simulink library "experiment_lib2"  (Simulink 8.3)
settings: Solver=ode45  SolverMode=SingleTasking  StartTime=0.0  StopTime=10.0  RelTol=1e-3
values from neighbouring files (symbols this model uses):
  kernel_drift = [0.05 0.05 0.05 0.05]    [Pau_Pol_6_Nodes_4_Perd_0_TxRate_0.01.mat]    (also in llencadora_sim.m = ones(1,num_generators)*0.1-0.05)
  kernel_offset = [0 0 0 0]    [Pau_Pol_6_Nodes_4_Perd_0_TxRate_0.01.mat]    (also in llencadora_sim.m = zeros(1,num_generators))
  LL = [0.000782892151765 0.000588394714514 0.000709966836418 0.00082261967749]    [Pau_Pol_6_Nodes_4_Perd_0_TxRate_0.01.mat]    (also in llencadora_sim.m = minLL+(maxLL-minLL)*rand(1,num_loads))
  Lline = [1.0827664502e-05 1.06430432216e-05 1.0255354423e-05 1.05299829153e-05]    [Pau_Pol_6_Nodes_4_Perd_0_TxRate_0.01.mat]    (also in llencadora_sim.m = minLline+(maxLline-minLline)*rand(1,num_lines))
  RL = [0.345490722943 0.282580500651 0.390474448437 0.324054882207]    [Pau_Pol_6_Nodes_4_Perd_0_TxRate_0.01.mat]    (also in llencadora_sim.m = minRL+(maxRL-minRL)*rand(1,num_loads))
  RLa_pos = 0.45    [Pau_Pol_6_Nodes_4_Perd_0_TxRate_0.01.mat]    (also in llencadora_sim.m = maxRL*ones(1,num_loads_act)*4/tot)
  RLa_pre = 0.21    [Pau_Pol_6_Nodes_4_Perd_0_TxRate_0.01.mat]    (also in llencadora_sim.m = minRL*ones(1,num_loads_act)*4/tot)
  Rline = [0.00149363403679 0.00820725625814 0.00655593060546 0.00272568602759]    [Pau_Pol_6_Nodes_4_Perd_0_TxRate_0.01.mat]    (also in llencadora_sim.m = minRline+(maxRline-minRline)*rand(1,num_lines))
  tL = 5    [Pau_Pol_6_Nodes_4_Perd_0_TxRate_0.01.mat]    (also in llencadora_sim.m = 1e10*ones(1,num_loads_act))
  ts = 0.0001    [Pau_Pol_6_Nodes_4_Perd_0_TxRate_0.01.mat]    (also in dintegral_w_code.m; llencadora_sim.m; processor.m = data.ts)
undefined symbols (not defined in the file or in its folder): CL
libraries: powerlib x17, simulink x1, truetime x1
settings Model: Creator=SEPIC  LastModifiedBy=mvelasco

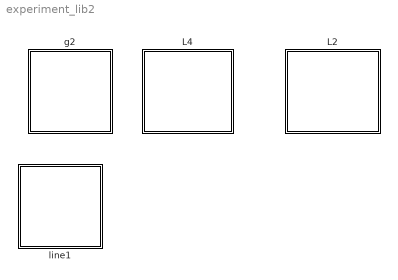
== system experiment_lib2 ==
  L2 : Subsystem  mask{a=1}
      mask Display: disp(['Active\nLoad\n' num2str(a)])
  L4 : Subsystem  mask{a=1}
      mask Display: disp(['Load\nLine\n' num2str(a)])
  g2 : Subsystem  RequirementInfo="{}  %GIDa_067657de_e0d2_47a1_a8cf_e324e59bc421"  mask{a=1}
      mask Display: disp(['Gen\nCom\n' num2str(a)]);
  line1 : Subsystem  mask{a=1}
      mask Display: disp(['Line\n' num2str(a)]);

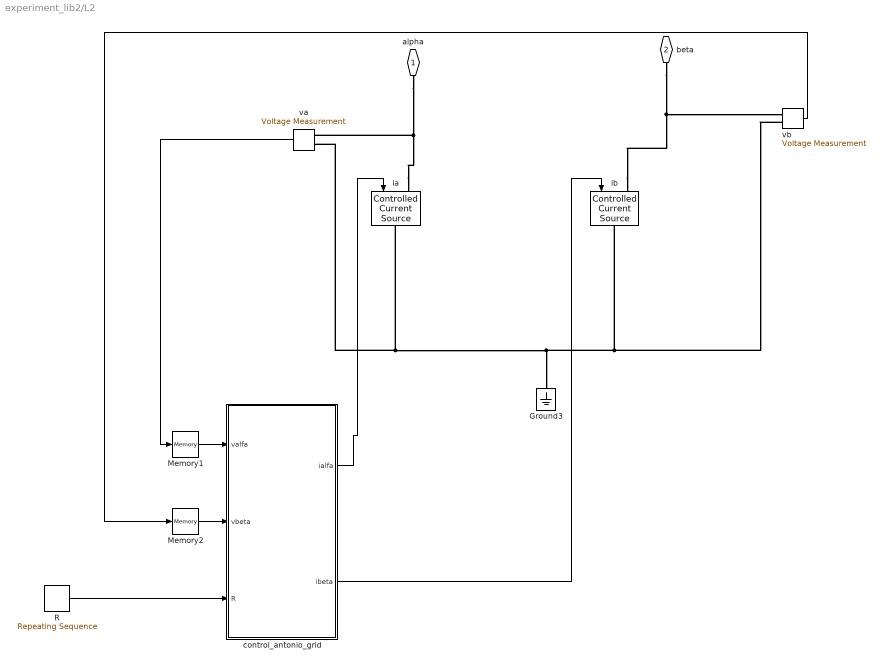
== system experiment_lib2/L2 ==
  Ground3 : powerlib/Elements/Ground  LConnTagsString=a
  Memory1 : Memory
  Memory2 : Memory
  R : simulink/Sources/Repeating Sequence  rep_seq_t=[0 tL(a) tL(a)+ts 1000]  rep_seq_y="[RLa_pre(a)  RLa_pre(a)  RLa_pos(a)  RLa_pos(a) ]"
  control_antonio_grid : MATLAB Function  TreatAsAtomicUnit=on
  ia : powerlib/Electrical Sources/Controlled Current Source  Initialize=on  Source_Type=AC  Amplitude=0  Phase=0  Frequency=0  Measurements=None
  ib : powerlib/Electrical Sources/Controlled Current Source  Initialize=on  Source_Type=AC  Amplitude=0  Phase=0  Frequency=0  Measurements=None
  va : powerlib/Measurements/Voltage Measurement  PhasorSimulation=off  OutputType=Complex  PSBequivalent=0
  vb : powerlib/Measurements/Voltage Measurement  PhasorSimulation=off  OutputType=Complex  PSBequivalent=0
  "alpha " : PMIOPort  Port=1  Side=Left
  beta : PMIOPort  Port=2  Side=Left
  wires:
  R/1 -> control_antonio_grid/3(R)
  va/1 -> Memory1/1
  vb/1 -> Memory2/1
  control_antonio_grid/1(ialfa) -> ia/1
  control_antonio_grid/2(ibeta) -> ib/1
  Memory1/1 -> control_antonio_grid/1(valfa)
  Memory2/1 -> control_antonio_grid/2(vbeta)
  connections:
  vb/LConn2 -- ib/RConn1 -- Ground3/LConn1 -- ia/RConn1 -- va/LConn2
  ia/LConn1 -- "alpha "/RConn1 -- va/LConn1
  ib/LConn1 -- beta/RConn1 -- vb/LConn1

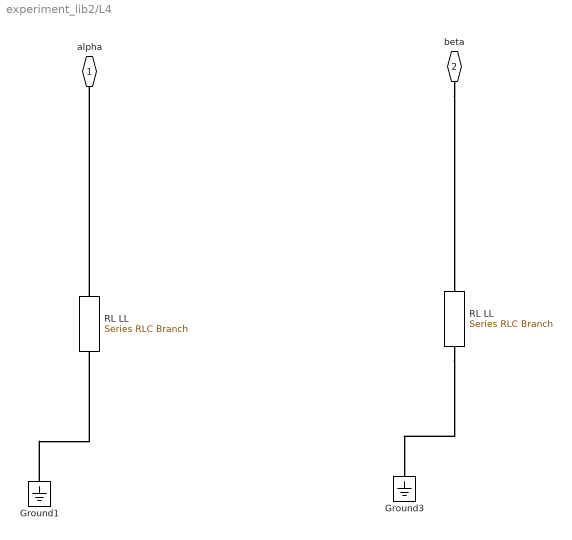
== system experiment_lib2/L4 ==
  Ground1 : powerlib/Elements/Ground  LConnTagsString=a
  Ground3 : powerlib/Elements/Ground  LConnTagsString=a
  RL LL : powerlib/Elements/Series RLC Branch  LConnTagsString=__new0  RConnTagsString=__new0  BranchType=RL  Resistance=RL(a)  Inductance=LL(a)  SetiL0=off  InitialCurrent=0  Capacitance=CL  Setx0=off  InitialVoltage=0  Measurements=None
  "RL LL   " : powerlib/Elements/Series RLC Branch  LConnTagsString=__new0  RConnTagsString=__new0  BranchType=RL  Resistance=RL(a)  Inductance=LL(a)  SetiL0=off  InitialCurrent=0  Capacitance=CL  Setx0=off  InitialVoltage=0  Measurements=None
  "alpha " : PMIOPort  Port=1  Side=Left
  beta : PMIOPort  Port=2  Side=Left
  connections:
  "RL LL   "/RConn1 -- Ground3/LConn1
  beta/RConn1 -- "RL LL   "/LConn1
  Ground1/LConn1 -- RL LL/RConn1
  RL LL/LConn1 -- "alpha "/RConn1

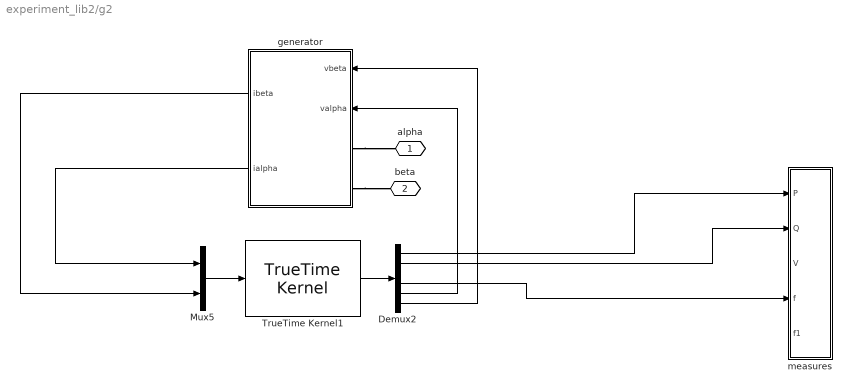
== system experiment_lib2/g2 ==
  Demux2 : Demux  Outputs=6
  Mux5 : Mux  Inputs=2
  TrueTime Kernel1 : truetime/TrueTime Kernel  sfun=kernel_init  args=[a]  ninputsoutputs=[2 6]  ntriggers=0  trigtype=falling  nwnodenbr=[1 a]  clockoffsetdrift=[kernel_offset(a) kernel_drift(a)]  schedoutput=off  battery=off  poweroutput=off
  generator : Subsystem
  measures : Subsystem
  alpha : PMIOPort  Port=1  Side=Left
  beta : PMIOPort  Port=2  Side=Left
  wires:
  generator/2("ialpha ") -> Mux5/1
  generator/1("ibeta ") -> Mux5/2
  Mux5/1 -> TrueTime Kernel1/1
  TrueTime Kernel1/1 -> Demux2/1
  Demux2/6 -> generator/1("vbeta  ")
  Demux2/5 -> generator/2("valpha ")
  Demux2/1 -> measures/1(P)
  Demux2/4 -> measures/4(f)
  Demux2/2 -> measures/2(Q)
  connections:
  generator/LConn1 -- alpha/RConn1
  generator/LConn2 -- beta/RConn1

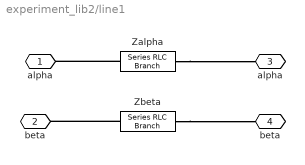
== system experiment_lib2/line1 ==
  Zalpha : powerlib/Elements/Series RLC Branch  LConnTagsString=__new0  RConnTagsString=__new0  BranchType=RL  Resistance=Rline(a)  Inductance=Lline(a)  SetiL0=off  InitialCurrent=0  Capacitance=CL  Setx0=off  InitialVoltage=0  Measurements=None
  Zbeta : powerlib/Elements/Series RLC Branch  LConnTagsString=__new0  RConnTagsString=__new0  BranchType=RL  Resistance=Rline(a)  Inductance=Lline(a)  SetiL0=off  InitialCurrent=0  Capacitance=CL  Setx0=off  InitialVoltage=0  Measurements=None
  alpha : PMIOPort  Port=1  Side=Left
  "beta " : PMIOPort  Port=2  Side=Left
  "alpha " : PMIOPort  Port=3  Side=Right
  "beta   " : PMIOPort  Port=4  Side=Right
  connections:
  Zbeta/RConn1 -- "beta "/RConn1
  Zbeta/LConn1 -- "beta   "/RConn1
  Zalpha/RConn1 -- alpha/RConn1
  Zalpha/LConn1 -- "alpha "/RConn1

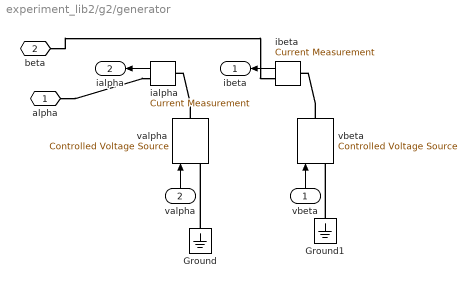
== system experiment_lib2/g2/generator ==
  "vbeta  " : Inport
  "valpha " : Inport  Port=2
  Ground : powerlib/Elements/Ground  LConnTagsString=a
  Ground1 : powerlib/Elements/Ground  LConnTagsString=a
  ialpha : powerlib/Measurements/Current Measurement  PhasorSimulation=off  OutputType=Complex  PSBequivalent=0
  ibeta : powerlib/Measurements/Current Measurement  PhasorSimulation=off  OutputType=Complex  PSBequivalent=0
  valpha : powerlib/Electrical Sources/Controlled Voltage Source  Initialize=on  Source_Type=AC  Amplitude=0  Phase=0  Frequency=0  Measurements=None
  vbeta : powerlib/Electrical Sources/Controlled Voltage Source  Initialize=on  Source_Type=AC  Amplitude=0  Phase=0  Frequency=0  Measurements=None
  alpha : PMIOPort  Port=1  Side=Left
  beta : PMIOPort  Port=2  Side=Left
  "ibeta " : Outport
  "ialpha " : Outport  Port=2
  wires:
  ialpha/1 -> "ialpha "/1
  ibeta/1 -> "ibeta "/1
  "valpha "/1 -> valpha/1
  "vbeta  "/1 -> vbeta/1
  connections:
  Ground/LConn1 -- valpha/LConn1
  Ground1/LConn1 -- vbeta/LConn1
  valpha/RConn1 -- ialpha/LConn1
  alpha/RConn1 -- ialpha/RConn1
  vbeta/RConn1 -- ibeta/LConn1
  beta/RConn1 -- ibeta/RConn1

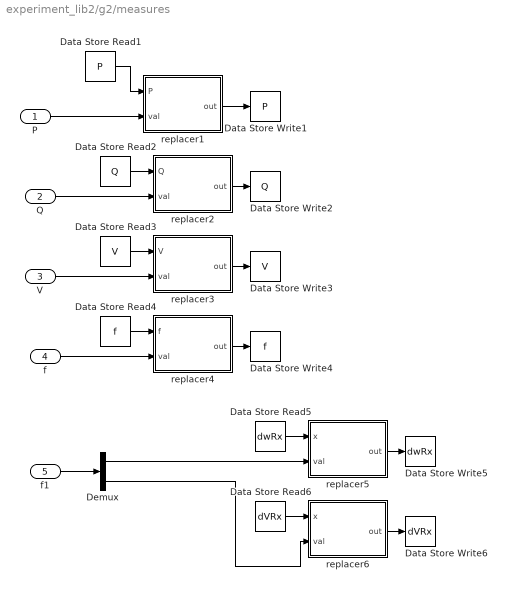
== system experiment_lib2/g2/measures ==
  P : Inport
  Q : Inport  Port=2
  V : Inport  Port=3
  f : Inport  Port=4
  f1 : Inport  Port=5
  Data Store Read1 : DataStoreRead  DataStoreName=P  SampleTime=0
  Data Store Read2 : DataStoreRead  DataStoreName=Q  SampleTime=0
  Data Store Read3 : DataStoreRead  DataStoreName=V  SampleTime=0
  Data Store Read4 : DataStoreRead  DataStoreName=f  SampleTime=0
  Data Store Read5 : DataStoreRead  DataStoreName=dwRx  SampleTime=0
  Data Store Read6 : DataStoreRead  DataStoreName=dVRx  SampleTime=0
  Data Store Write1 : DataStoreWrite  DataStoreName=P
  Data Store Write2 : DataStoreWrite  DataStoreName=Q
  Data Store Write3 : DataStoreWrite  DataStoreName=V
  Data Store Write4 : DataStoreWrite  DataStoreName=f
  Data Store Write5 : DataStoreWrite  DataStoreName=dwRx
  Data Store Write6 : DataStoreWrite  DataStoreName=dVRx
  Demux : Demux  Outputs=2
  replacer1 : MATLAB Function  TreatAsAtomicUnit=on
  replacer2 : MATLAB Function  TreatAsAtomicUnit=on
  replacer3 : MATLAB Function  TreatAsAtomicUnit=on
  replacer4 : MATLAB Function  TreatAsAtomicUnit=on
  replacer5 : MATLAB Function  TreatAsAtomicUnit=on
  replacer6 : MATLAB Function  TreatAsAtomicUnit=on
  wires:
  replacer2/1(out) -> Data Store Write2/1
  Data Store Read2/1 -> replacer2/1(Q)
  replacer3/1(out) -> Data Store Write3/1
  Data Store Read3/1 -> replacer3/1(V)
  replacer4/1(out) -> Data Store Write4/1
  Data Store Read4/1 -> replacer4/1(f)
  Q/1 -> replacer2/2(val)
  V/1 -> replacer3/2(val)
  f/1 -> replacer4/2(val)
  f1/1 -> Demux/1
  replacer5/1(out) -> Data Store Write5/1
  replacer6/1(out) -> Data Store Write6/1
  Data Store Read6/1 -> replacer6/1(x)
  Data Store Read5/1 -> replacer5/1(x)
  Demux/1 -> replacer5/2(val)
  Demux/2 -> replacer6/2(val)
  Data Store Read1/1 -> replacer1/1(P)
  replacer1/1(out) -> Data Store Write1/1
  P/1 -> replacer1/2(val)

== matlab function g2/measures/replacer1 ==
  settings: updateMethod=DISCRETE  sampleTime=data_rate
  data: P input double; out output double; val input double; a parameter double
function out  = fcn2(P,val,a)
out=P;
out(a)=val;

== matlab function g2/measures/replacer2 ==
  settings: updateMethod=DISCRETE  sampleTime=data_rate
  data: Q input double; out output double; val input double; a parameter double
function out  = fcn2(Q,val,a)
out=Q;
out(a)=val;

== matlab function g2/measures/replacer3 ==
  settings: updateMethod=DISCRETE  sampleTime=data_rate
  data: V input double; out output double; val input double; a parameter double
function out  = fcn2(V,val,a)
out=V;
out(a)=val;

== matlab function g2/measures/replacer4 ==
  settings: updateMethod=DISCRETE  sampleTime=data_rate
  data: f input double; out output double; val input double; a parameter double
function out  = fcn2(f,val,a)
out=f;
out(a)=val;

== matlab function g2/measures/replacer5 ==
  settings: updateMethod=DISCRETE  sampleTime=data_rate
  data: x input double; out output double; val input double; a parameter double
function out  = fcn2(x,val,a)
out=x;
out(a)=val;

== matlab function g2/measures/replacer6 ==
  settings: updateMethod=DISCRETE  sampleTime=data_rate
  data: x input double; out output double; val input double; a parameter double
function out  = fcn2(x,val,a)
out=x;
out(a)=val;

== matlab function L2/control_antonio_grid ==
  data: valfa input double size=1; ialfa output double; vbeta input double; R input double; ibeta output double
function [ialfa,ibeta]= fcn7(valfa, vbeta, R)

ialfa=valfa/R;
ibeta=vbeta/R;
